simulink model "batt_test"  (Simulink 7.8)
settings: Solver=ode3  StartTime=0.0  StopTime=20  FixedStep=80e-6  RelTol=1e-3
PostLoadFcn:
  | Ts=80e-6;
InitFcn:
  | Ts=80e-6;
values from neighbouring files (symbols this model uses):
  batt_esr = (max_power*0.01)/(max_power/Vdc_nom)^2    [BES_init.m]
  C = IacRMS*18e-6    [BES_init.m]
  f = 60    [global_parameters.m]
  I_ki = 0.03    [BES_init.m]
  I_kp = 0.05    [BES_init.m]
  Iac_max = IGBT_currents(possible_currents(1))    [BES_init.m]
  Id_at_max = 3*max_pow*(2/3)/Vd_at_max    [BES_init.m]
  Iq_at_max = 3*max_pow*(2/3)/Vq_at_max    [BES_init.m]
  L = Vdc_nom/(IacRMS*0.2/(2/fs))    [BES_init.m]
  PLL_Ki = 0.001*30    (= 0.03)    [BES_init.m]
  PLL_Kp = .001*30    (= 0.03)    [BES_init.m]
  PLL_time_step = Ts    (= 8e-05)    [global_parameters.m]
  Roff = 1e7    (= 10000000)    [BES_init.m]
  Td_es_min = Ts    (= 8e-05)    [global_parameters.m]
  Tds = Ts    (= 8e-05)    [global_parameters.m]
  Vdc_max = IGBT_voltages(possible_voltages(1))    [BES_init.m]
undefined symbols (not defined in the file or in its folder): D, DiscIntNeverNeededParam
libraries: simulink x25, powerlib x20, simulink_extras x10, cstextras x9, powerlib_extras x8, modbus_lib x6, dynamic_load_lib x1, dspsigops x1
(part 1 of 2)
settings Model: Creator=ch24070  LastModifiedBy=ch24070

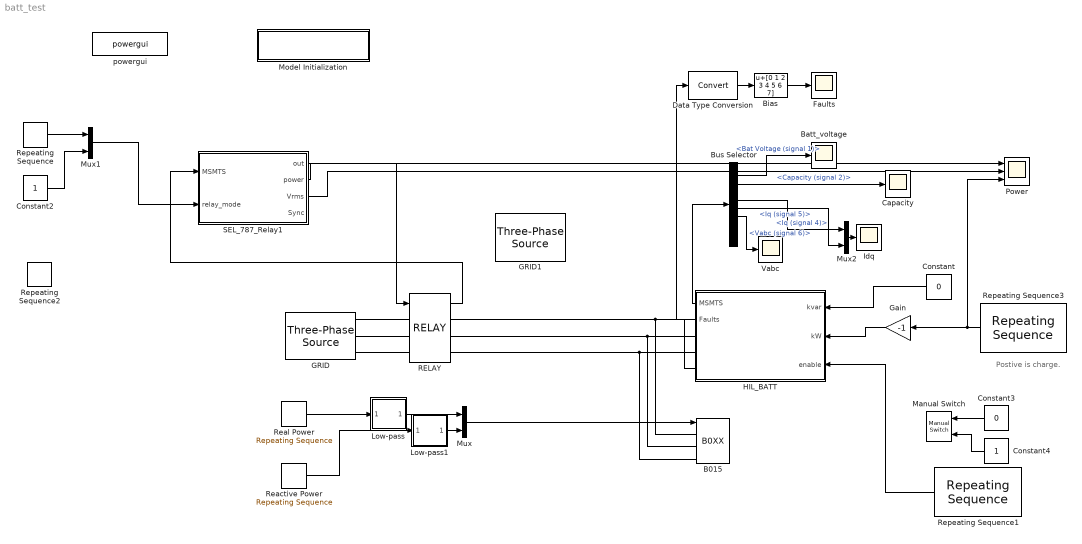
== system batt_test ==
  note: Postive is charge.
  B015 : dynamic_load_lib/B0XX  V=2047  P_Scale=1  Q_Scale=1
  Batt_voltage : Scope
      settings: YMin=500  YMax=4250  SaveName=ScopeData3
  Bias : Bias  Bias=[0 1 2 3 4 5 6 7]
  Bus Selector : BusSelector  OutputSignals=Bat Voltage (signal 1),Capacity (signal 2),Batt Iout (signal 3),Iq (signal 4),Iq (signal 5),Vabc (signal 6),Iabc (signal 7),freq (signal 8)
  Capacity : Scope
      settings: YMin=-0.05  YMax=1.05  SaveName=ScopeData4
  Constant : Constant  Value=0
  Constant2 : Constant
  Constant3 : Constant  Value=0
  Constant4 : Constant
  Data Type Conversion : DataTypeConversion
  Faults : Scope
      settings: TimeRange=10  YMin=0  YMax=10
  GRID : powerlib/Electrical Sources/Three-Phase Source  Voltage=2078  PhaseAngle=0  Frequency=60  InternalConnection=Yg  SpecifyImpedance=on  Resistance=0.8929  Inductance=16.58e-3  ShortCircuitLevel=375e6  BaseVoltage=2078  XRratio=7.9  BusType=swing  Pref=0  Qref=0  Qmin=-inf  Qmax=inf
  GRID1 : powerlib/Electrical Sources/Three-Phase Source  Voltage=1  PhaseAngle=0  Frequency=60*5  InternalConnection=Yg  SpecifyImpedance=on  Resistance=0.8929  Inductance=16.58e-3  ShortCircuitLevel=375e3  BaseVoltage=2078  XRratio=7.9  BusType=swing  Pref=0  Qref=0  Qmin=-inf  Qmax=inf
  Gain : Gain  Gain=-1
  HIL_BATT : Subsystem
  Idq : Scope
      settings: YMin=-1750  YMax=1750  SaveName=ScopeData6
  Low-pass : Subsystem  BlockChoice=CSS  mask(LTI Block){sys=c2d(tf(1,[1/(1*2*pi),1]),Ts), IC=[]}
      mask prompts: sys "LTI system variable"; IC "Initial states (state-space only)"
      mask help:
      | The LTI System block accepts both continuous and discrete LTI models as defined in the Control System Toolbox. Transfer function, state-space, and zero-pole-gain formats are all supported in this block.
      |
      | Note: Initial states are only meaningful for state-space systems.
      mask init:
      | try
      |    % read data to initialize mask variables
      |    [D,Ts,Tdi,Tdo,Tdio,x0,sysname]=...
      |       ltimask('Initialize',gcb,sys,IC);
      |    % update contents
      |    model = bdroot;
      |    df = get_param(model,'dirty');
      |    ltimask('UpdateDiagram',gcb,D,Ts,Tdio);
      |    try      
      |       % Attempt to modify locked library -> error
      |       % Makes block show ??? when loading CSTBLOCKS
      |       % for the first time
      |       set_param(model,'dirty',df)
      |    end
      | catch ME
      |    sys = [];  IC = [];   sysname = '???';
      |    throw(ME)
      | end
      mask Help:
      | The LTI System block accepts any of the three standard LTI models described in the Control System Toolbox: transfer function, zero/pole/gain, or state space. Internally, LTI models will be converted to their state space equivalent for evaluation.
      | <p>
      | In the editable text box labeled <b>LTI System Variable</b>, enter a valid LTI model.
      | <p>
      | In the editable text box labeled <b>Initial States</b> enter the initial state vector.  Initial states are only valid for state-space systems.
      | <p>
      | See also TF, ZPK, SS, LTIMODELS.
      mask CallbackString: ltimask('MaskLTICallback',gcb);|
      mask Display: disp(sysname)
  Low-pass1 : Subsystem  BlockChoice=CSS  mask(LTI Block){sys=c2d(tf(1,[1/(1*2*pi),1]),Ts), IC=[]}
      mask prompts: sys "LTI system variable"; IC "Initial states (state-space only)"
      mask help:
      | The LTI System block accepts both continuous and discrete LTI models as defined in the Control System Toolbox. Transfer function, state-space, and zero-pole-gain formats are all supported in this block.
      |
      | Note: Initial states are only meaningful for state-space systems.
      mask init: same as batt_test/Low-pass
      mask Help:
      | The LTI System block accepts any of the three standard LTI models described in the Control System Toolbox: transfer function, zero/pole/gain, or state space. Internally, LTI models will be converted to their state space equivalent for evaluation.
      | <p>
      | In the editable text box labeled <b>LTI System Variable</b>, enter a valid LTI model.
      | <p>
      | In the editable text box labeled <b>Initial States</b> enter the initial state vector.  Initial states are only valid for state-space systems.
      | <p>
      | See also TF, ZPK, SS, LTIMODELS.
      mask CallbackString: ltimask('MaskLTICallback',gcb);|
      mask Display: disp(sysname)
  Manual Switch : simulink/Signal Routing/Manual Switch  sw=1  action=0  varsize=off
  Model Initialization : Subsystem  AncestorBlock=artemis/Tools /Misc/Model Initialization  mask(Model Functions){InitFcnX=Ts=80e-6;, prel=off, posl=on, inif=on, strf=off}
      mask prompts: InitFcnX "Initialisation"; prel "Preload Function"; posl "PostLoad Function"; inif "InitFcn"; strf "StartFcn"
      mask init:
      | currentBlock = gcb;
      | root = bdroot(currentBlock);
      | 
      | if ~strcmp(get_param(root,'BlockDiagramType'),'library')
      |     if prel==1
      |         set_param(root, 'PreLoadFcn', InitFcnX);
      |     else
      |         set_param(root, 'PreLoadFcn', '');
      |     end
      |     if inif==1
      |         set_param(root, 'InitFcn', InitFcnX);
      |     else
      |         set_param(root, 'InitFcn', '');
      |     end
      |     if strf==1
      |         set_param(root, 'StartFcn', InitFcnX);
      |     else
      |         set_param(root, 'StartFcn', '');
      |     end
      |     if posl==1
      |         set_param(root, 'PostLoadFcn', InitFcnX);
      |     else
      |         set_param(root, 'PostLoadFcn', '');
      |     end
      | end
      | 
      | pos = get_param(currentBlock, 'Position');
      | width = pos(3) - pos(1); height = pos(4) - pos(2);
      | txt = [ upper(root) '\n' '- InitFcn. . . . . '  get_param(root, 'InitFcn') ];
      settings: CopyFcn=set_param(gcb,'LinkStatus','inactive')
      mask Display: text(5, height*0.5, txt, 'horizontalAlignment', 'left', 'verticalAlignment', 'middle') ;
  Mux : Mux  Inputs=2
  Mux1 : Mux  Inputs=2
  Mux2 : Mux  Inputs=2
  Power : Scope  NumInputPorts=3
      settings: YMin=-5000~0~3800  YMax=5000~1400~4200
  RELAY : modbus_lib/RELAY  Ts=Ts
      link override Three-Phase V-I Measurement/Model/VI/Ia: GotoTag=LibraryTag_Ia
      link override Three-Phase V-I Measurement/Model/VI/Ib: GotoTag=LibraryTag_Ib
      link override Three-Phase V-I Measurement/Model/VI/Ic: GotoTag=LibraryTag_Ic
      link override Three-Phase V-I Measurement/Model/VI/Va: GotoTag=LibraryTag_Va
      link override Three-Phase V-I Measurement/Model/VI/Vb: GotoTag=LibraryTag_Vb
      link override Three-Phase V-I Measurement/Model/VI/Vc: GotoTag=LibraryTag_Vc
      link override Three-Phase V-I Measurement1/Model/VI/Ia: GotoTag=LibraryTag_Ia
      link override Three-Phase V-I Measurement1/Model/VI/Ib: GotoTag=LibraryTag_Ib
      link override Three-Phase V-I Measurement1/Model/VI/Ic: GotoTag=LibraryTag_Ic
      link override Three-Phase V-I Measurement1/Model/VI/Va: GotoTag=LibraryTag_Va
      link override Three-Phase V-I Measurement1/Model/VI/Vb: GotoTag=LibraryTag_Vb
      link override Three-Phase V-I Measurement1/Model/VI/Vc: GotoTag=LibraryTag_Vc
  Reactive Power : simulink/Sources/Repeating Sequence  rep_seq_t=[0 2 4 6]  rep_seq_y=[0 50 0 50]
  Real Power : simulink/Sources/Repeating Sequence  rep_seq_t=[0 2 4 6]  rep_seq_y=[0 100 0 100]
  Repeating Sequence : simulink/Sources/Repeating Sequence  rep_seq_t=[0 2]  rep_seq_y=[0 0]
  Repeating Sequence1 : simulink/Sources/Repeating Sequence  rep_seq_t=[0 2 2 5 5 6 6 7 12]  rep_seq_y=[0 0 1 1 0 0 1 1 1]
  Repeating Sequence2 : simulink/Sources/Repeating Sequence  rep_seq_t=[0 3 3 5 5 6 7]  rep_seq_y=[0 0 2 2 1 1 0]
  Repeating Sequence3 : simulink/Sources/Repeating Sequence  rep_seq_t=[0 2 2 5 5 6 6 7 12]  rep_seq_y=4000.*[0 0 1 1 0 0 -1 -1 -1]
  SEL_787_Relay1 : Subsystem  mask{IOC=30000, TOC=2500, VRMSLL=13800, Ts=Ts}
      mask prompts: IOC "IOC Setting [A]"; TOC "TOC Setting [A]"; VRMSLL "Nominal Voltage [VRMSLL]"; Ts "Sampling Time [Sec]"
  Vabc : Scope
      settings: TimeRange=5.446467479375272e-005  YMin=-0.02823442247358754  YMax=0.1118314007674113  SaveName=ScopeData2
  powergui : powerlib/powergui  Priority=2  SimulationMode=Discrete  SolverType=Tustin  SampleTime=Ts  frequency=60  SPID=off  DisableSnubberDevices=off  DisableRonSwitches=off  DisableVfSwitches=off  SwTol=0  Interpol=off  DisplayEquations=off  FunctionMessages=off  frequencyindice=0  Pbase=100e6  ErrMax=1e-4  Iterations=50  UnitsV=kV  UnitsW=MW  echomessages=off  HookPort=off  EnableUseOfTLC=off  x0status=blocks  RestoreLinks=warning  ResistiveCurrentMeasurement=off  Frange=logspace(0,3,50)  Ylog=off  Xlog=off  ShowGrid=off  save=off  variable=ZData  structure=0  ZoomFFT=on  StartTime=0.0  cycles=2  DisplayStyle=off  fundamental=60  FreqAxis=off  MaxFrequency=1000  frequencyindicesteady=1  RmsSteady=1  display=off  Ts=0  methode=off
  wires:
  RELAY/1 -> SEL_787_Relay1/1(MSMTS)
  HIL_BATT/1(MSMTS) -> Bus Selector/1
  HIL_BATT/2(Faults) -> Data Type Conversion/1
  Constant/1 -> HIL_BATT/1(kvar)
  Repeating Sequence3/1 -> Gain/1, Power/3
  SEL_787_Relay1/1(out) -> RELAY/1
  SEL_787_Relay1/2(power) -> Power/1
  Bus Selector/6 -> Vabc/1  "<Vabc (signal 6)>"
  Bus Selector/1 -> Batt_voltage/1  "<Bat Voltage (signal 1)>"
  Bus Selector/2 -> Capacity/1  "<Capacity (signal 2)>"
  Gain/1 -> HIL_BATT/2(kW)
  Bias/1 -> Faults/1
  Data Type Conversion/1 -> Bias/1
  Mux/1 -> B015/1
  Real Power/1 -> Low-pass/1(In1)
  Reactive Power/1 -> Low-pass1/1(In1)
  Low-pass/1(Out1) -> Mux/1
  Low-pass1/1(Out1) -> Mux/2
  Mux1/1 -> SEL_787_Relay1/2(relay_mode)
  SEL_787_Relay1/3(Vrms) -> Power/2
  Repeating Sequence/1 -> Mux1/1
  Constant2/1 -> Mux1/2
  Constant3/1 -> Manual Switch/1
  Constant4/1 -> Manual Switch/2
  Mux2/1 -> Idq/1
  Bus Selector/4 -> Mux2/1  "<Iq (signal 4)>"
  Bus Selector/5 -> Mux2/2  "<Iq (signal 5)>"
  Repeating Sequence1/1 -> HIL_BATT/3(enable)
  connections:
  GRID/RConn2 -- RELAY/LConn2
  GRID/RConn1 -- RELAY/LConn1
  GRID/RConn3 -- RELAY/LConn3
  RELAY/RConn1 -- HIL_BATT/RConn1 -- B015/LConn1
  RELAY/RConn2 -- HIL_BATT/RConn2 -- B015/LConn2
  RELAY/RConn3 -- HIL_BATT/RConn3 -- B015/LConn3

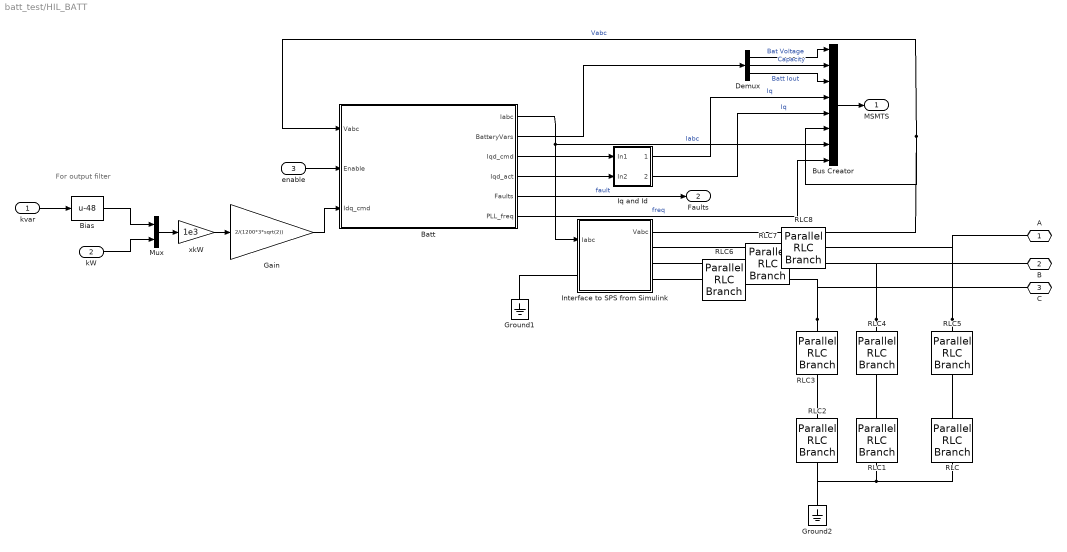
== system batt_test/HIL_BATT ==
  note: For output filter
  kvar : Inport
  kW : Inport  Port=2
  enable : Inport  Port=3
  Batt : Subsystem  mask(Battery Energy Storage System with AC inverter and Droop Control){max_power=4e6, batt_kWh=5, VacRMS=1200, Vdc_nom=4000}
      mask prompts: max_power "Peak Power (W)"; batt_kWh "Capacity (kWh)"; VacRMS "Grid Tie Line to Neutral Voltage (RMS)"; Vdc_nom "Nominal DC Battery Voltage"
      mask help: The block implements a battery energy storage system suitable for connecting to the grid. It responds to grid voltage changes by injecting current into the grid. The model is a non-switching average model.
      mask init:
      | global_parameters
      | BES_init
      mask Help:
      | This block will likely need a filter and transformer on it's output in order to connect to a high power line.
      | 
      | A unit delay block  on the Iabc output can help remove algebraic loops with minimal impact on simulation results.
      | 
      | 
      | Block Parameters:
      | Peak Power- Maximum power the unit can transfer.
      | Capacity- Amount of energy in the battery.
      | Grid Tie Line to Neutral Voltage- RMS voltage for the grid tie interface.
      | Nominal DC Battery Voltage- Open circuit full charge voltage.
      | Real Power Droop Gain- Ratio of Watts to Hz for injecting power to the grid in response to frequency changes.
      | Reactive Power Droop Gain- Ratio of kVars to RMS volts for injecting reactive power to the grid.
      | Droop Filter Cut Off- Fastest frequency that will be responded to for injecting power to the grid.
      | 
      | 
      | Block Connections:
      | Vabc- Grid voltage for each of the three phases.
      | Enable- Set to zero for no power.  Set to 1 to enable energy tranfer.
      | Iabc- Grid current for each of the three phases.  Connect to your grid.  Positive is into the grid.
      | Battery_vars- A vector of battery voltage, capacity, and current out of the battery.
      | Iqd_cmd- Commanded q and d axis currents.
      | Iqd_act- Actual q and d axis currents.
      mask Display:
      | image(imread('grid_storage_battery.jpg'))
      | color('white')
      | fprintf('%d kW Peak', max_power/1e3)
      | color('black')
      | port_label('input',1,'Vabc')
      | port_label('input',2,'Enable')
      | port_label('input',3,'Idq_cmd')
      | port_label('output',1,'Iabc')
      | port_label('output',2,'Battery_vars')
      | port_label('output',3,'Iqd_cmd')
      | port_label('output',4,'Iqd_act')
      | port_label('output',5,'Faults')
      | port_label('output',6,'Freq')
  Bias : Bias  Bias=-48
  Bus Creator : BusCreator  Inputs=8
  Demux : Demux  Outputs=3
  Gain : Gain  Gain=2/(1200*3*sqrt(2))
  Ground1 : powerlib/Elements/Ground  LConnTagsString=a
  Ground2 : powerlib/Elements/Ground  LConnTagsString=a
  Interface to SPS from Simulink : Subsystem
  Iq and Id : Subsystem
  Mux : Mux  Inputs=2
  "RLC " : powerlib/Elements/Parallel RLC Branch  LConnTagsString=a  RConnTagsString=__new0  BranchType=RLC  Resistance=500  Inductance=inf  SetiL0=off  InitialCurrent=0  Capacitance=10e-6  Setx0=off  InitialVoltage=0  Measurements=None
  RLC1 : powerlib/Elements/Parallel RLC Branch  LConnTagsString=a  RConnTagsString=__new0  BranchType=RLC  Resistance=500  Inductance=inf  SetiL0=off  InitialCurrent=0  Capacitance=10e-6  Setx0=off  InitialVoltage=0  Measurements=None
  RLC2 : powerlib/Elements/Parallel RLC Branch  LConnTagsString=a  RConnTagsString=__new0  BranchType=RLC  Resistance=500  Inductance=inf  SetiL0=off  InitialCurrent=0  Capacitance=10e-6  Setx0=off  InitialVoltage=0  Measurements=None
  RLC3 : powerlib/Elements/Parallel RLC Branch  LConnTagsString=a  RConnTagsString=__new0  BranchType=R  Resistance=10e-3  Inductance=inf  SetiL0=off  InitialCurrent=0  Capacitance=0  Setx0=off  InitialVoltage=0  Measurements=None
  RLC4 : powerlib/Elements/Parallel RLC Branch  LConnTagsString=a  RConnTagsString=__new0  BranchType=R  Resistance=10e-3  Inductance=inf  SetiL0=off  InitialCurrent=0  Capacitance=0  Setx0=off  InitialVoltage=0  Measurements=None
  RLC5 : powerlib/Elements/Parallel RLC Branch  LConnTagsString=a  RConnTagsString=__new0  BranchType=R  Resistance=10e-3  Inductance=inf  SetiL0=off  InitialCurrent=0  Capacitance=0  Setx0=off  InitialVoltage=0  Measurements=None
  RLC6 : powerlib/Elements/Parallel RLC Branch  LConnTagsString=a  RConnTagsString=__new0  BranchType=R  Resistance=20e-3  Inductance=inf  SetiL0=off  InitialCurrent=0  Capacitance=0  Setx0=off  InitialVoltage=0  Measurements=None
  RLC7 : powerlib/Elements/Parallel RLC Branch  LConnTagsString=a  RConnTagsString=__new0  BranchType=R  Resistance=20e-3  Inductance=inf  SetiL0=off  InitialCurrent=0  Capacitance=0  Setx0=off  InitialVoltage=0  Measurements=None
  RLC8 : powerlib/Elements/Parallel RLC Branch  LConnTagsString=a  RConnTagsString=__new0  BranchType=R  Resistance=20e-3  Inductance=inf  SetiL0=off  InitialCurrent=0  Capacitance=0  Setx0=off  InitialVoltage=0  Measurements=None
  xkW : Gain  Gain=1e3
  A : PMIOPort  Port=1  Side=Right
  B : PMIOPort  Port=2  Side=Right
  C : PMIOPort  Port=3  Side=Right
  MSMTS : Outport
  Faults : Outport  Port=2
  wires:
  Bias/1 -> Mux/1
  Batt/6(PLL_freq) -> Bus Creator/8  "freq"
  kW/1 -> Mux/2
  kvar/1 -> Bias/1
  Bus Creator/1 -> MSMTS/1
  Iq and Id/2(Out2) -> Bus Creator/5  "Iq"
  Mux/1 -> xkW/1
  xkW/1 -> Gain/1
  Gain/1 -> Batt/3(Idq_cmd)
  Batt/1(Iabc) -> Interface to SPS from Simulink/1(Iabc), Bus Creator/7  "Iabc"
  enable/1 -> Batt/2(Enable)
  Iq and Id/1(Out1) -> Bus Creator/4  "Iq"
  Batt/4(Iqd_act) -> Iq and Id/2(In2)
  Batt/3(Iqd_cmd) -> Iq and Id/1(In1)
  Demux/1 -> Bus Creator/1  "Bat Voltage"
  Demux/3 -> Bus Creator/3  "Batt Iout"
  Demux/2 -> Bus Creator/2  "Capacity"
  Batt/2(BatteryVars) -> Demux/1
  Interface to SPS from Simulink/1(Vabc) -> Bus Creator/6, Batt/1(Vabc)  "Vabc"
  Batt/5(Faults) -> Faults/1  "fault"
  connections:
  Interface to SPS from Simulink/RConn1 -- RLC8/RConn1
  Interface to SPS from Simulink/RConn2 -- RLC7/RConn1
  RLC6/RConn1 -- Interface to SPS from Simulink/RConn3
  RLC5/RConn1 -- "RLC "/LConn1
  RLC4/RConn1 -- RLC1/LConn1
  RLC3/RConn1 -- RLC2/LConn1
  RLC3/LConn1 -- RLC6/LConn1 -- C/RConn1
  RLC4/LConn1 -- RLC7/LConn1 -- B/RConn1
  RLC5/LConn1 -- RLC8/LConn1 -- A/RConn1
  RLC1/RConn1 -- "RLC "/RConn1 -- RLC2/RConn1 -- Ground2/LConn1
  Interface to SPS from Simulink/LConn1 -- Ground1/LConn1

== system batt_test/Low-pass ==
  In1 : Inport
  IO Delay : cstextras/Integer Delay (masked)  Td=Tdio  u0=0  Ts=Ts
  Input Delay : cstextras/Integer Delay (masked)  Td=Tdi  u0=0  Ts=Ts
  Internal : DiscreteStateSpace  A=D.a  B=D.b  C=D.c  D=D.d  SampleTime=Ts
  Output Delay : cstextras/Integer Delay (masked)  Td=Tdo  u0=0  Ts=Ts
  Out1 : Outport  InitialOutput=0
  wires:
  In1/1 -> Input Delay/1
  Output Delay/1 -> Out1/1
  Input Delay/1 -> Internal/1
  Internal/1 -> IO Delay/1
  IO Delay/1 -> Output Delay/1

== system batt_test/Low-pass1 ==
  In1 : Inport
  IO Delay : cstextras/Integer Delay (masked)  Td=Tdio  u0=0  Ts=Ts
  Input Delay : cstextras/Integer Delay (masked)  Td=Tdi  u0=0  Ts=Ts
  Internal : DiscreteStateSpace  A=D.a  B=D.b  C=D.c  D=D.d  SampleTime=Ts
  Output Delay : cstextras/Integer Delay (masked)  Td=Tdo  u0=0  Ts=Ts
  Out1 : Outport  InitialOutput=0
  wires:
  In1/1 -> Input Delay/1
  Output Delay/1 -> Out1/1
  Input Delay/1 -> Internal/1
  Internal/1 -> IO Delay/1
  IO Delay/1 -> Output Delay/1

== system batt_test/Model Initialization ==

== system batt_test/SEL_787_Relay1 ==
  MSMTS : Inport
  relay_mode : Inport  Port=2
  Bus Creator : BusCreator  Inputs=3
  Bus Selector1 : BusSelector  OutputSignals=Iabc,Vabc_bus,Vabc_line
  Bus Selector2 : BusSelector  OutputSignals=signal19,signal20,signal10
  Mux : Mux  Inputs=2
  SEL_787_Relay : Subsystem  AncestorBlock=modbus_lib/SEL_787_Relay  mask(SEL_787){bkrCtrl_enable=0, bkrCtrl_status=1}
      mask prompts: bkrCtrl_enable "Enable - manual breaker control"; bkrCtrl_status "Status - manual breaker control"
      mask help:
      | Reynaldo Ulerio
      | Jason LaPenta
      | Aidan Dowdle
      | Matt Backes
      | Sept 14, 2015
      | ________________________________
      |
      | Based off the SEL-787 transformer relay, this model receives
      | the three-phase current and voltage measurements, and packs
      | them along with other calculations to send to the microgrid
      | controller via Modbus
      |
      | - See HIL packet for detailed list of signals and scale factors
      | - Follows convention of IEEE C37.2-2008
      |
      | Procedure to reclose a breaker:
      | 1) reset all relay functions
      | 2) set orvvp_mode==1 to force breaker to close
      |    --> The relay function 25 will automatically activate
      | 3) change op_mode==0 for logic based operation
      |
      | * Additional and for debuging: Allows the user to select which trip signal will be received at the breaker.
      |
      | Manual breaker status: [1-closed, 0-open]
  out : Outport
  power : Outport  Port=2
  Vrms : Outport  Port=3
  Sync : Outport  Port=4
  wires:
  SEL_787_Relay/1(op_mode) -> Bus Creator/1  "op_mode"
  SEL_787_Relay/2(Logic_trip) -> Bus Creator/2  "Logic_trip"
  SEL_787_Relay/3(m) -> Bus Creator/3  "m"
  SEL_787_Relay/4(TO_MODBUS) -> Bus Selector2/1
  Bus Creator/1 -> out/1  "SEL_787_Relay1"
  MSMTS/1 -> Bus Selector1/1
  Bus Selector1/1 -> SEL_787_Relay/1(Iabc)  "<Iabc>"
  Bus Selector1/2 -> SEL_787_Relay/2(Vabc_bus)  "<Vabc_bus>"
  Bus Selector1/3 -> SEL_787_Relay/3(Vabc_line)  "<Vabc_line>"
  Bus Selector2/1 -> Mux/1  "<signal19>"
  Bus Selector2/2 -> Mux/2  "<signal20>"
  Mux/1 -> power/1
  relay_mode/1 -> SEL_787_Relay/4(FROM_MODBUS)
  Bus Selector2/3 -> Vrms/1  "<signal10>"
  SEL_787_Relay/5(Sync) -> Sync/1

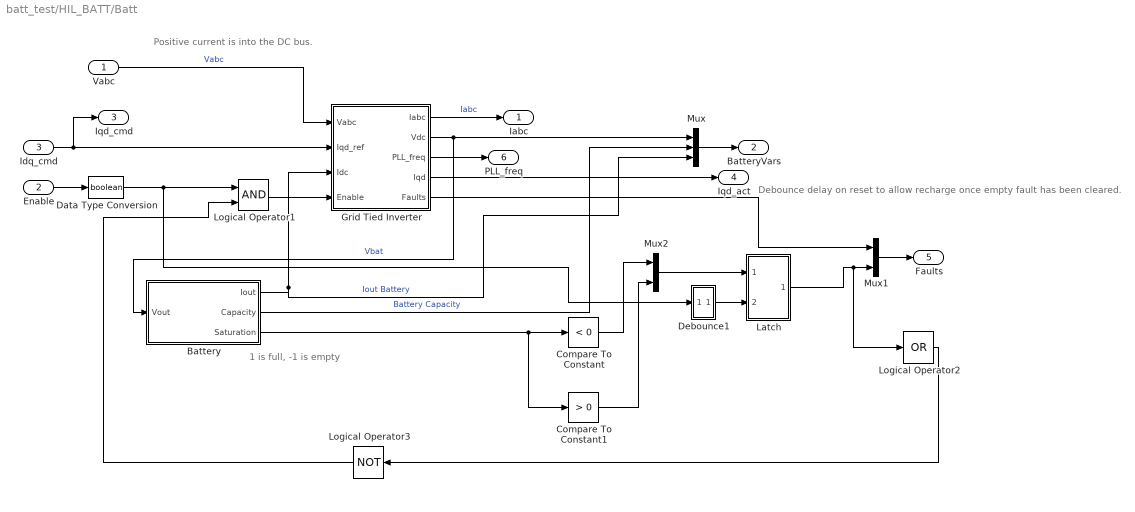
== system batt_test/HIL_BATT/Batt ==
  note: Positive current is into the DC bus.
  note: 1 is full, -1 is empty
  note: Debounce delay on reset to allow recharge once empty fault has been cleared.
  Vabc : Inport
  Enable : Inport  Port=2  OutDataTypeStr=double
  Idq_cmd : Inport  Port=3
  Battery : Subsystem  mask(Very simple battery model.  ){kWh=batt_kWh, esr=batt_esr, Vdc_nom=Vdc_nom}
      mask prompts: kWh "Capacity  (kWh)"; esr "Output Resistance (Ohms)"; Vdc_nom "Open Circuit Voltage"
      mask help: Model integrates charge and stops at the rated capacity. When charge is all removed the current drops to zero.
      mask Help: This model views the battery as a voltage source with a fixed equivalent series resistance and a perfect integrator for capacity.
  Compare To Constant : simulink/Logic and Bit Operations/Compare To Constant  relop=<  const=0  OutDataTypeStr=boolean
  Compare To Constant1 : simulink/Logic and Bit Operations/Compare To Constant  relop=>  const=0  OutDataTypeStr=boolean
  Data Type Conversion : DataTypeConversion  OutDataTypeStr=boolean
  Debounce1 : Subsystem  mask{Ts=Ts, Td=0.1}
      mask prompts: Ts "Sample Time"; Td "Debounce Time"
  Grid Tied Inverter : Subsystem
  Latch : Subsystem
  Logical Operator1 : Logic  AllPortsSameDT=off  OutDataTypeStr=boolean
  Logical Operator2 : Logic  Operator=OR  Inputs=1  AllPortsSameDT=off  OutDataTypeStr=boolean
  Logical Operator3 : Logic  Operator=NOT  AllPortsSameDT=off  OutDataTypeStr=boolean
  Mux : Mux  Inputs=3
  Mux1 : Mux  Inputs=2
  Mux2 : Mux  Inputs=2
  Iabc : Outport
  BatteryVars : Outport  Port=2
  Iqd_cmd : Outport  Port=3
  Iqd_act : Outport  Port=4
  Faults : Outport  Port=5
  PLL_freq : Outport  Port=6
  wires:
  Grid Tied Inverter/3(PLL_freq) -> PLL_freq/1
  Vabc/1 -> Grid Tied Inverter/1(Vabc)  "Vabc"
  Grid Tied Inverter/2(Vdc) -> Mux/1, Battery/1(Vout)  "Vbat"
  Battery/1(Iout) -> Grid Tied Inverter/3(Idc), Mux/3  "Iout Battery"
  Battery/2(Capacity) -> Mux/2  "Battery Capacity"
  Grid Tied Inverter/1(Iabc) -> Iabc/1  "Iabc"
  Mux/1 -> BatteryVars/1
  Grid Tied Inverter/4(Iqd) -> Iqd_act/1
  Idq_cmd/1 -> Grid Tied Inverter/2(Iqd_ref), Iqd_cmd/1
  Enable/1 -> Data Type Conversion/1
  Mux1/1 -> Faults/1
  Battery/3(Saturation) -> Compare To Constant/1, Compare To Constant1/1
  Compare To Constant/1 -> Mux2/1
  Compare To Constant1/1 -> Mux2/2
  Logical Operator1/1 -> Grid Tied Inverter/4(Enable)
  Data Type Conversion/1 -> Logical Operator1/1, Debounce1/1(In1)
  Logical Operator2/1 -> Logical Operator3/1
  Logical Operator3/1 -> Logical Operator1/2
  Grid Tied Inverter/5(Faults) -> Mux1/1
  Latch/1(Out1) -> Mux1/2, Logical Operator2/1
  Mux2/1 -> Latch/1(In1)
  Debounce1/1(Out1) -> Latch/2(Reset)

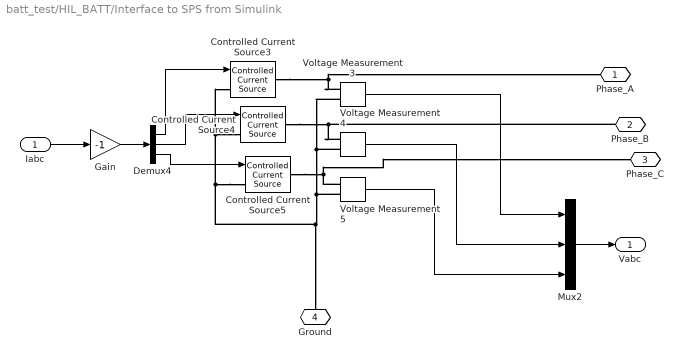
== system batt_test/HIL_BATT/Interface to SPS from Simulink ==
  Iabc : Inport
  Controlled Current Source3 : powerlib/Electrical Sources/Controlled Current Source  Initialize=on  Source_Type=AC  Amplitude=0  Phase=0  Frequency=0  Measurements=None
  Controlled Current Source4 : powerlib/Electrical Sources/Controlled Current Source  Initialize=on  Source_Type=AC  Amplitude=0  Phase=0  Frequency=0  Measurements=None
  Controlled Current Source5 : powerlib/Electrical Sources/Controlled Current Source  Initialize=on  Source_Type=AC  Amplitude=0  Phase=0  Frequency=0  Measurements=None
  Demux4 : Demux  Outputs=3
  Gain : Gain  Gain=-1
  Mux2 : Mux  Inputs=3
  Voltage Measurement3 : powerlib/Measurements/Voltage Measurement  PhasorSimulation=off  OutputType=Complex  PSBequivalent=0
  Voltage Measurement4 : powerlib/Measurements/Voltage Measurement  PhasorSimulation=off  OutputType=Complex  PSBequivalent=0
  Voltage Measurement5 : powerlib/Measurements/Voltage Measurement  PhasorSimulation=off  OutputType=Complex  PSBequivalent=0
  Phase_A : PMIOPort  Port=1  Side=Right
  Phase_B : PMIOPort  Port=2  Side=Right
  Phase_C : PMIOPort  Port=3  Side=Right
  Ground : PMIOPort  Port=4  Side=Left
  Vabc : Outport
  wires:
  Voltage Measurement5/1 -> Mux2/3
  Voltage Measurement4/1 -> Mux2/2
  Demux4/1 -> Controlled Current Source3/1
  Demux4/2 -> Controlled Current Source4/1
  Demux4/3 -> Controlled Current Source5/1
  Iabc/1 -> Gain/1
  Mux2/1 -> Vabc/1
  Voltage Measurement3/1 -> Mux2/1
  Gain/1 -> Demux4/1
  connections:
  Voltage Measurement5/LConn1 -- Controlled Current Source5/RConn1 -- Phase_C/RConn1
  Voltage Measurement3/LConn1 -- Controlled Current Source3/RConn1 -- Phase_A/RConn1
  Controlled Current Source5/LConn1 -- Controlled Current Source3/LConn1 -- Controlled Current Source4/LConn1 -- Voltage Measurement4/LConn2 -- Voltage Measurement3/LConn2 -- Voltage Measurement5/LConn2 -- Ground/RConn1
  Voltage Measurement4/LConn1 -- Controlled Current Source4/RConn1 -- Phase_B/RConn1

== system batt_test/HIL_BATT/Iq and Id ==
  In1 : Inport
  In2 : Inport  Port=2
  Demux1 : Demux  Outputs=2
  Demux2 : Demux  Outputs=2
  Mux : Mux  Inputs=2
  Mux1 : Mux  Inputs=2
  Out1 : Outport
  Out2 : Outport  Port=2
  wires:
  Mux1/1 -> Out2/1
  Mux/1 -> Out1/1
  In2/1 -> Demux2/1
  In1/1 -> Demux1/1
  Demux2/2 -> Mux1/2  "Id_act"
  Demux1/1 -> Mux/1  "Iq_cmd"
  Demux2/1 -> Mux/2  "Iq_act"
  Demux1/2 -> Mux1/1  "Id_cmd"

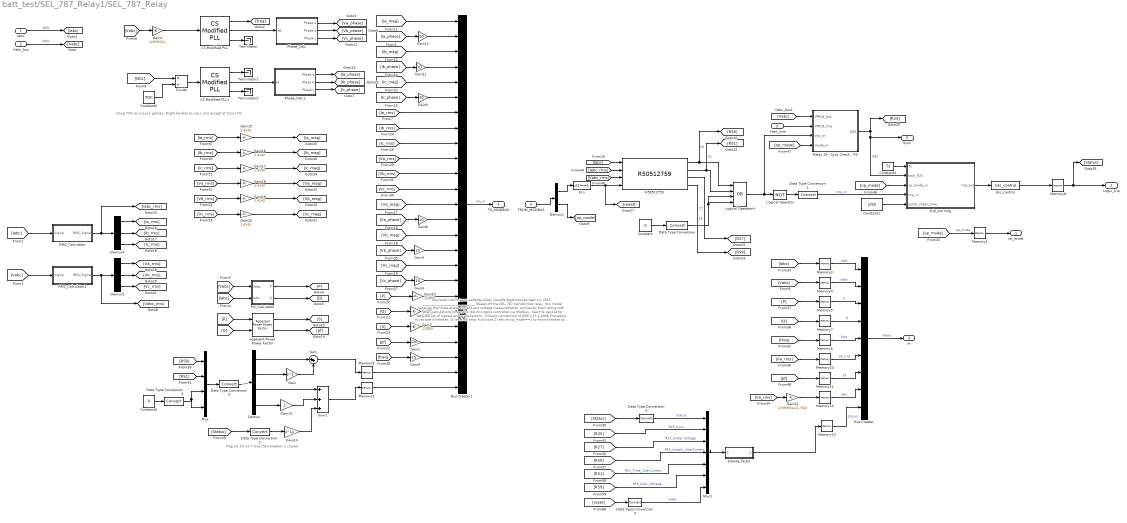
== system batt_test/SEL_787_Relay1/SEL_787_Relay ==
  note: Reg 24: bit 14 = true then breaker is closed
  note: Using TOC as a quick getway. Might be able to use I_rms except at time t=0.
  note: Reynaldo Ulerio
      | Jason LaPenta
      | Aidan Dowdle
      | Matt Backes
      | Sept 14, 2015
      | ________________________________
      |
      | Based off the SEL-787 transformer relay, this model receives
      | the three-phase current and voltage measurements, and packs
      | them along with other calculations to send to the microgrid
      | controller via Modbus
      |
      | - See HIL packet for detailed list of signals and scale factors
      | - Follows convention of IEEE C37.2-2008
      |
      | Procedure to reclose a breaker:
      | 1) reset all relay functions
      | 2) set orvvp_mode==1 to force breaker to close
      |    --> The relay function 25 will automatically activate
      | 3) change op_mode==0 for logic based operation
  Iabc : Inport
  Vabc_bus : Inport  Port=2
  Vabc_line : Inport  Port=3
  FROM_MODBUS : Inport  Port=4
  Apparent Power Power Factor : modbus_lib/Apparent Power Power Factor
  Bus Creator : BusCreator  Inputs=9
  Bus Creator1 : BusCreator  Inputs=25
  CS Modified PLL : modbus_lib/CS Modified PLL  Fmin=50  Par_Init=[0 60]  ParK=[ 180 3200 1 ]  Ts=Ts  AGC=off
  CS Modified PLL1 : modbus_lib/CS Modified PLL  Fmin=50  Par_Init=[0 60]  ParK=[ 180 3200 1 ]  Ts=Ts  AGC=off
  Constant : Constant  Value=0
  Constant1 : Constant  Value=2/60
  Constant2 : Constant  Value=TOC
  Constant3 : Constant  Value=0
  Constant4 : Constant  Value=Ts
  Data Type Conversion{,1..6} (7 alike) : DataTypeConversion
  Demux : Demux
  Demux2 : Demux  Outputs=2
  Demux4 : Demux  Outputs=3
  Demux5 : Demux  Outputs=3
  Divide : Product  Inputs=*/
  Fcn : Fcn  Expr=u(1)==1
  Gain : Gain  Gain=2^3
  Gain1 : Gain  Gain=100
  Gain10 : Gain  Gain=1/1000
  Gain{3..5,8..9,11..12} (7 alike) : Gain  Gain=10
  Gain13 : Gain  Gain=2
  Gain14 : Gain  Gain=2^14
  Gain{15..20} (6 alike) : Gain  Gain=1.4142
  Gain2 : Gain  Gain=1/VRMSLL
  Gain21 : Gain  Gain=1/(VRMSLL/1.732)
  Gain6 : Gain  Gain=1/1000
  Gain7 : Gain  Gain=1/1000
  Logical Operator : Logic  Operator=NOT  AllPortsSameDT=off  OutDataTypeStr=boolean
  Logical Operator4 : Logic  Operator=OR  Inputs=4  AllPortsSameDT=off  OutDataTypeStr=boolean
  Memory{1..13} (13 alike) : Memory
  Mux : Mux
  Mux1 : Mux  Inputs=7
  PQ_Calculator : Subsystem
  Phase_Calc : Subsystem
  Phase_Calc1 : Subsystem
  R50512759 : modbus_lib/R50512759  VRMSLL=VRMSLL  IOC=IOC  TOC=TOC  Ts=Ts
  RMS_Calculator : Subsystem
  RMS_Calculator1 : Subsystem
  Relay 25 - Sync Check - RS : Subsystem  AncestorBlock=modbus_lib/Relay 25 - Sync Check - RS  mask{VRMSLL=VRMSLL, Ts=Ts}
      mask prompts: VRMSLL "Nominal Voltage [VRMSLL]"; Ts "Sampling Time [Sec]"
  Sum : Sum  Inputs=|++
  Sum1 : Sum  Inputs=+++
  Terminator : Terminator
  Terminator1 : Terminator
  Terminator2 : Terminator
  bitwise_faults : Subsystem
  bkr_control : modbus_lib/bkr_control  enable=bkrCtrl_enable  status=bkrCtrl_status
  trip_out mng : MATLAB Function  TreatAsAtomicUnit=on
  op_mode : Outport
  Logic_trip : Outport  Port=2
  m : Outport  Port=3
  TO_MODBUS : Outport  Port=4
  Sync : Outport  Port=5
  wires:
  Data Type Conversion6/1 -> Mux1/1  "Status"
  Data Type Conversion5/1 -> Mux1/7  "reset"
  [R59] -> Mux1/6  "R59_Over_Voltage"
  [R51] -> Mux1/5  "R51_Time_OverCurrent"
  [R50] -> Mux1/4  "R50_Instant_OverCurrent"
  [R27] -> Mux1/3  "R27_Under Voltage"
  [R25] -> Mux1/2  "R25_Sync"
  [Status] -> Data Type Conversion6/1
  [reset] -> Data Type Conversion5/1
  bitwise_faults/1(s) -> Memory13/1
  Mux1/1 -> bitwise_faults/1(S)
  Data Type Conversion3/1 -> Mux/4, Mux/3
  Constant3/1 -> Data Type Conversion3/1
  R50512759/4 -> [R59]  "59"
  R50512759/3 -> [R27]  "27"
  Data Type Conversion/1 -> Logical Operator4/3, Logical Operator4/4
  Constant/1 -> Data Type Conversion/1
  bkr_control/1 -> Memory8/1
  Bus Creator/1 -> m/1  "meas"
  Memory13/1 -> Bus Creator/9  "status"
  Apparent Power Power Factor/2 -> [pf]
  Apparent Power Power Factor/1 -> [S]
  Constant4/1 -> trip_out mng/1(Ts)
  Gain21/1 -> Memory12/1
  Memory12/1 -> Bus Creator/8  "Vpu"
  [Va_rms] -> Gain21/1
  Gain15/1 -> [Ia_mag]
  Gain16/1 -> [Ib_mag]
  Gain17/1 -> [Ic_mag]
  Gain18/1 -> [Va_mag]
  Gain19/1 -> [Vb_mag]
  Gain20/1 -> [Vc_mag]
  [Vc_rms] -> Gain20/1
  [Vb_rms] -> Gain19/1
  [Va_rms] -> Gain18/1
  [Ic_rms] -> Gain17/1
  [Ib_rms] -> Gain16/1
  [Ia_rms] -> Gain15/1
  Vabc_bus/1 -> [Vabc]  "Vabc"
  Vabc_line/1 -> Relay 25 - Sync Check - RS/2(VPKLN_line)
  [Vabc] -> Relay 25 - Sync Check - RS/1(VPKLN_bus)
  [Status] -> Data Type Conversion2/1
  Gain14/1 -> Sum1/3
  Data Type Conversion2/1 -> Gain14/1
  Gain4/1 -> Bus Creator1/23
  Gain1/1 -> Bus Creator1/22
  Gain7/1 -> Bus Creator1/21
  Gain6/1 -> Bus Creator1/20
  Gain10/1 -> Bus Creator1/19
  Gain3/1 -> Bus Creator1/18
  [Vc_mag] -> Bus Creator1/17
  Gain5/1 -> Bus Creator1/16
  [Vb_mag] -> Bus Creator1/15
  Gain8/1 -> Bus Creator1/14
  [Va_mag] -> Bus Creator1/13
  [Vc_rms] -> Bus Creator1/12
  [Vb_rms] -> Bus Creator1/11
  [Va_rms] -> Bus Creator1/10
  [Ic_rms] -> Bus Creator1/9
  [Ib_rms] -> Bus Creator1/8
  [Ia_rms] -> Bus Creator1/7
  Gain9/1 -> Bus Creator1/6
  [Ic_mag] -> Bus Creator1/5
  Gain11/1 -> Bus Creator1/4
  [Ib_mag] -> Bus Creator1/3
  Gain12/1 -> Bus Creator1/2
  [Ia_mag] -> Bus Creator1/1
  Memory11/1 -> Bus Creator/7  "pf"
  [pf] -> Memory11/1
  Memory10/1 -> Bus Creator/6  "Va_rms"
  Memory6/1 -> Bus Creator/5  "freq"
  [Va_rms] -> Memory10/1
  [freq] -> Memory6/1
  CS Modified PLL/3 -> Terminator/1
  CS Modified PLL1/3 -> Terminator2/1
  CS Modified PLL1/1 -> Terminator1/1
  CS Modified PLL/2 -> Phase_Calc/1(wt)
  CS Modified PLL/1 -> [freq]
  CS Modified PLL1/2 -> Phase_Calc1/1(wt)
  trip_out mng/1(trip_out) -> bkr_control/1
  [op_mode] -> Relay 25 - Sync Check - RS/4(mode_in)
  Data Type Conversion1/1 -> trip_out mng/4(trip_in)  "trip_in"
  [op_mode] -> trip_out mng/3(op_mode_in)
  Relay 25 - Sync Check - RS/1(R25) -> [R25], trip_out mng/2(bool_R25), Sync/1  "R25"
  Constant1/1 -> trip_out mng/5(synch_check_time)
  Memory8/1 -> [Status], Logic_trip/1
  Memory1/1 -> op_mode/1
  [op_mode] -> Memory1/1  "op_mode"
  Fcn/1 -> [reset], R50512759/4
  [Iabc_rms] -> R50512759/2
  Memory7/1 -> Bus Creator/4  "Q"
  Memory5/1 -> Bus Creator/3  "P"
  Memory4/1 -> Bus Creator/2  "Vabc"
  Memory3/1 -> Bus Creator/1  "Iabc"
  Memory2/1 -> Bus Creator1/25
  Memory9/1 -> Bus Creator1/24
  Data Type Conversion4/1 -> Demux/1
  Demux/4 -> Gain13/1
  Demux/3 -> Sum1/1
  Demux/2 -> Gain/1
  Demux/1 -> Sum/1
  Mux/1 -> Data Type Conversion4/1
  [R51] -> Mux/2
  [R50] -> Mux/1
  R50512759/2 -> [R51], Logical Operator4/2  "51"
  Gain/1 -> Sum/2
  Sum/1 -> Memory9/1
  Gain13/1 -> Sum1/2
  Sum1/1 -> Memory2/1
  R50512759/1 -> [R50], Logical Operator4/1  "50"
  Logical Operator/1 -> Data Type Conversion1/1
  Logical Operator4/1 -> Relay 25 - Sync Check - RS/3(trip_or), Logical Operator/1
  [Vabc_rms] -> R50512759/3
  [Ia_phase] -> Gain12/1
  [Ib_phase] -> Gain11/1
  [Ic_phase] -> Gain9/1
  [Va_phase] -> Gain8/1
  [Vb_phase] -> Gain5/1
  [Vc_phase] -> Gain3/1
  Constant2/1 -> Divide/2
  Divide/1 -> CS Modified PLL1/1
  Phase_Calc1/3(Phase c) -> [Ic_phase]
  Phase_Calc1/2(Phase b) -> [Ib_phase]
  Phase_Calc1/1(Phase a) -> [Ia_phase]
  [Iabc] -> Divide/1
  Phase_Calc/3(Phase c) -> [Vc_phase]
  Phase_Calc/2(Phase b) -> [Vb_phase]
  Phase_Calc/1(Phase a) -> [Va_phase]
  Gain2/1 -> CS Modified PLL/1
  [Vabc] -> Gain2/1
  [Q] -> Memory7/1
  [P] -> Memory5/1
  [pf] -> Gain1/1
  [freq] -> Gain4/1
  Bus Creator1/1 -> TO_MODBUS/1  "sm_in"
  FROM_MODBUS/1 -> Demux2/1
  [Vabc] -> Memory4/1
  [Iabc] -> Memory3/1
  Iabc/1 -> [Iabc]  "Iabc"
  [Vabc] -> PQ_Calculator/1(Vabc)
  [Iabc] -> PQ_Calculator/2(Iabc)
  [P] -> Gain10/1
  [Q] -> Gain6/1
  [S] -> Gain7/1
  [P] -> Apparent Power Power Factor/1
  [Q] -> Apparent Power Power Factor/2
  PQ_Calculator/1(P) -> [P]
  PQ_Calculator/2(Q) -> [Q]
  [Iabc] -> RMS_Calculator/1(Signal)
  [Vabc] -> RMS_Calculator1/1(Signal)
  RMS_Calculator/1(RMS_Signal) -> [Iabc_rms], Demux4/1
  RMS_Calculator1/1(RMS_Signal) -> [Vabc_rms], Demux5/1
  Demux4/3 -> [Ic_rms]
  Demux4/2 -> [Ib_rms]
  Demux4/1 -> [Ia_rms]
  Demux5/1 -> [Va_rms]
  Demux5/2 -> [Vb_rms]
  Demux5/3 -> [Vc_rms]
  Demux2/1 -> Fcn/1
  [Iabc] -> R50512759/1
  Demux2/2 -> [op_mode]

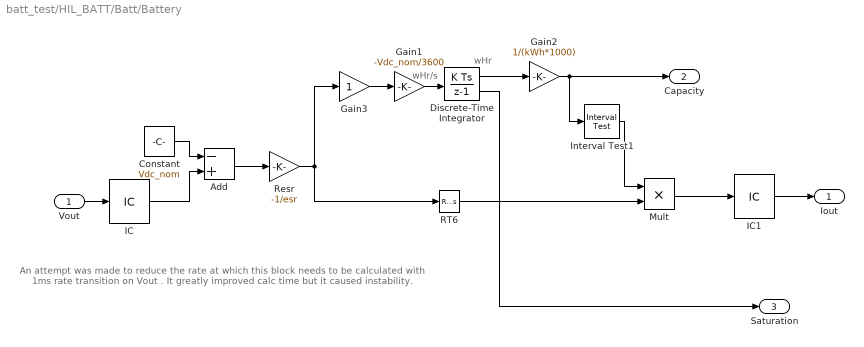
== system batt_test/HIL_BATT/Batt/Battery ==
  note: An attempt was made to reduce the rate at which this block
      | needs to be calculated with 1ms rate transition on
      | Vout .  It greatly improved calc time but it caused instability.
  note: wHr/s
  note: wHr
  Vout : Inport
  Add : Sum  Inputs=-+
  Constant : Constant  Value=Vdc_nom  SampleTime=Tds
  Discrete-Time Integrator : DiscreteIntegrator  InitialCondition=kWh*0.5*1000  InitialConditionMode=State only (most efficient)  SampleTime=Tds  LimitOutput=on  UpperSaturationLimit=(kWh*1000)  LowerSaturationLimit=0  ShowSaturationPort=on  ICPrevOutput=DiscIntNeverNeededParam  ICPrevScaledInput=DiscIntNeverNeededParam
  Gain1 : Gain  Gain=-Vdc_nom/3600
  Gain2 : Gain  Gain=1/(kWh*1000)
  Gain3 : Gain
  IC : InitialCondition  Value=Vdc_nom
  IC1 : InitialCondition  Value=0
  Interval Test1 : simulink/Logic and Bit Operations/Interval Test  IntervalClosedRight=on  uplimit=1  IntervalClosedLeft=on  lowlimit=0  OutDataTypeStr=boolean
  Mult : Product  Inputs=**
  RT6 : RateTransition  OutPortSampleTime=Tds
  Resr : Gain  Gain=-1/esr
  Iout : Outport
  Capacity : Outport  Port=2
  Saturation : Outport  Port=3
  wires:
  Constant/1 -> Add/1
  Add/1 -> Resr/1
  Gain1/1 -> Discrete-Time Integrator/1
  Interval Test1/1 -> Mult/1
  Vout/1 -> IC/1
  Mult/1 -> IC1/1
  Resr/1 -> RT6/1, Gain3/1
  Gain2/1 -> Capacity/1, Interval Test1/1
  Discrete-Time Integrator/1 -> Gain2/1
  IC/1 -> Add/2
  IC1/1 -> Iout/1
  RT6/1 -> Mult/2
  Gain3/1 -> Gain1/1
  Discrete-Time Integrator/2 -> Saturation/1

== system batt_test/HIL_BATT/Batt/Debounce1 ==
  In1 : Inport
  Compare To Constant1 : simulink/Logic and Bit Operations/Compare To Constant  relop=>  const=1  OutDataTypeStr=boolean
  Discrete-Time Integrator : DiscreteIntegrator  IntegratorMethod=Accumulation: Forward Euler  gainval=Ts/Td  ExternalReset=level  SampleTime=Ts  OutDataTypeStr=double  UpperSaturationLimit=1.001  LowerSaturationLimit=0  ICPrevOutput=DiscIntNeverNeededParam  ICPrevScaledInput=DiscIntNeverNeededParam
  Logical Operator : Logic  Operator=NOT  AllPortsSameDT=off  OutDataTypeStr=boolean
  Out1 : Outport
  wires:
  Compare To Constant1/1 -> Out1/1
  In1/1 -> Discrete-Time Integrator/1, Logical Operator/1
  Logical Operator/1 -> Discrete-Time Integrator/2
  Discrete-Time Integrator/1 -> Compare To Constant1/1

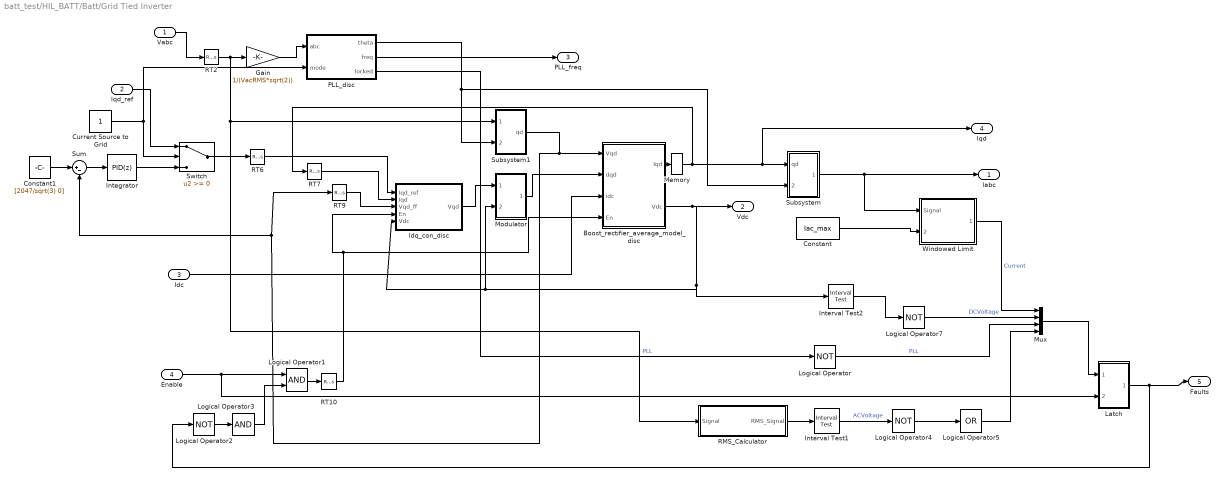
== system batt_test/HIL_BATT/Batt/Grid Tied Inverter ==
  Vabc : Inport
  Iqd_ref : Inport  Port=2
  Idc : Inport  Port=3
  Enable : Inport  Port=4
  Boost_rectifier_average_model_disc : Subsystem  mask{C=C, L=L, Roff=Roff, Vdc_nom=Vdc_nom}
      mask prompts: C "DC Bus Capacitance"; L "Boost Inductor"; Roff "Switch resistance when off"; Vdc_nom "Nominal DC Bus Voltage"
      mask init:
      | global_parameters
  Constant : Constant  Value=Iac_max
  Constant1 : Constant  Value=[2047/sqrt(3) 0]
  Current Source to Grid : Constant
  Gain : Gain  Gain=1/(VacRMS*sqrt(2))
  Idq_con_disc : Subsystem  mask{L=L, iq_max=Iq_at_max, id_max=Id_at_max, kp=I_kp, ki=I_ki, Vdc_nom=Vdc_nom}
      mask prompts: L "Boost Inductor"; iq_max "Maximum Iq"; id_max "Maximum Id"; kp "Proportional Gain"; ki "Integral Gain"; Vdc_nom "Nominal DC Bus Voltage"
      mask init:
      | global_parameters
  Integrator : simulink/Continuous/PID Controller  Controller=PID  TimeDomain=Discrete-time  SampleTime=Ts  IntegratorMethod=Forward Euler  FilterMethod=Forward Euler  Form=Parallel  P=2  I=0  D=0  N=100  InitialConditionSource=internal  InitialConditionForIntegrator=0  InitialConditionForFilter=0  ExternalReset=none  LimitOutput=on  UpperSaturationLimit=2000  LowerSaturationLimit=-2000  LinearizeAsGain=off  AntiWindupMode=clamping  Kb=1  TrackingMode=off  Kt=1  PParamMin=[]  PParamMax=[]  IParamMin=[]  IParamMax=[]  DParamMin=[]  DParamMax=[]  NParamMin=[]  NParamMax=[]  KbParamMin=[]  KbParamMax=[]  KtParamMin=[]  KtParamMax=[]  POutMin=[]  POutMax=[]  IOutMin=[]  IOutMax=[]  DOutMin=[]  DOutMax=[]  NOutMin=[]  NOutMax=[]  KbOutMin=[]  KbOutMax=[]  KtOutMin=[]  KtOutMax=[]  IntegratorOutMin=[]  IntegratorOutMax=[]  FilterOutMin=[]  FilterOutMax=[]  SumOutMin=[]  SumOutMax=[]  SumI1OutMin=[]  SumI1OutMax=[]  SumI2OutMin=[]  SumI2OutMax=[]  SumI3OutMin=[]  SumI3OutMax=[]  SumDOutMin=[]  SumDOutMax=[]  SaturationOutMin=[]  SaturationOutMax=[]  IntegratorContinuousStateAttributes=''  IntegratorStateMustResolveToSignalObject=off  IntegratorRTWStateStorageClass=Auto  FilterContinuousStateAttributes=''  FilterStateMustResolveToSignalObject=off  FilterRTWStateStorageClass=Auto
  Interval Test1 : simulink/Logic and Bit Operations/Interval Test  IntervalClosedRight=on  uplimit=VacRMS*1.1  IntervalClosedLeft=on  lowlimit=VacRMS*0.9  OutDataTypeStr=boolean
  Interval Test2 : simulink/Logic and Bit Operations/Interval Test  IntervalClosedRight=on  uplimit=Vdc_max  IntervalClosedLeft=on  lowlimit=2000  OutDataTypeStr=boolean
  Latch : Subsystem
  Logical Operator{,2,4,7} (4 alike) : Logic  Operator=NOT  AllPortsSameDT=off  OutDataTypeStr=boolean
  Logical Operator1 : Logic  AllPortsSameDT=off  OutDataTypeStr=boolean
  Logical Operator3 : Logic  Inputs=1  AllPortsSameDT=off  OutDataTypeStr=boolean
  Logical Operator5 : Logic  Operator=OR  Inputs=1  AllPortsSameDT=off  OutDataTypeStr=boolean
  Memory : Memory  InheritSampleTime=on
  Modulator : Subsystem
  Mux : Mux
  PLL_disc : Subsystem  mask{PLL_Kp=PLL_Kp, PLL_Ki=PLL_Ki, PLL_freq_range=0.25, PLL_lock_window=0.1}
      mask prompts: PLL_Kp "Proportional Gain"; PLL_Ki "Integral Gain"; PLL_freq_range "PLL Frequency Range"; PLL_lock_window "PLL Lock Window"
  RMS_Calculator : Subsystem
  RT{2,6..7,9..10} (5 alike) : RateTransition  OutPortSampleTime=Td_es_min
  Subsystem : Subsystem
  Subsystem1 : Subsystem
  Sum : Sum  Inputs=|+-
  Switch : Switch
  Windowed Limit : Subsystem
  Iabc : Outport
  Vdc : Outport  Port=2
  PLL_freq : Outport  Port=3
  Iqd : Outport  Port=4
  Faults : Outport  Port=5
  wires:
  Latch/1(Out1) -> Faults/1, Logical Operator2/1
  Mux/1 -> Latch/1(In1)
  RT7/1 -> Idq_con_disc/2(Iqd)
  Idc/1 -> Boost_rectifier_average_model_disc/3(idc)
  Boost_rectifier_average_model_disc/2(Vdc) -> Modulator/2(Vdc), Idq_con_disc/5(Vdc), Interval Test2/1, Vdc/1
  Logical Operator5/1 -> Mux/4
  Logical Operator4/1 -> Logical Operator5/1
  Interval Test1/1 -> Logical Operator4/1  "ACVoltage"
  RMS_Calculator/1(RMS_Signal) -> Interval Test1/1
  Logical Operator3/1 -> Logical Operator1/2
  Logical Operator2/1 -> Logical Operator3/1
  Subsystem1/1(qd) -> Boost_rectifier_average_model_disc/1(Vqd), RT9/1, Sum/2
  Boost_rectifier_average_model_disc/1(Iqd) -> Memory/1
  Subsystem/1(abc) -> Windowed Limit/1(Signal), Iabc/1
  Idq_con_disc/1(Vqd) -> Modulator/1(Vqd)
  Logical Operator1/1 -> RT10/1
  Constant/1 -> Windowed Limit/2(Threshold)
  Windowed Limit/1(TestOut) -> Mux/1  "Current"
  Interval Test2/1 -> Logical Operator7/1
  PLL_disc/2(freq) -> PLL_freq/1
  Modulator/1(dqd) -> Boost_rectifier_average_model_disc/2(dqd)
  PLL_disc/3(locked) -> Logical Operator/1  "PLL"
  Logical Operator/1 -> Mux/3  "PLL"
  Gain/1 -> PLL_disc/1(abc)
  Enable/1 -> Logical Operator1/1, Latch/2(Reset)
  PLL_disc/1(theta) -> Subsystem1/2(theta), Subsystem/2(theta)
  Vabc/1 -> RT2/1
  RT2/1 -> RMS_Calculator/1(Signal), Subsystem1/1(abc), Gain/1
  RT6/1 -> Idq_con_disc/1(Iqd_ref)
  RT9/1 -> Idq_con_disc/3(Vqd_ff)
  RT10/1 -> Boost_rectifier_average_model_disc/4(En), Idq_con_disc/4(En)
  Memory/1 -> Subsystem/1(qd), Iqd/1, RT7/1
  Logical Operator7/1 -> Mux/2  "DCVoltage"
  Switch/1 -> RT6/1
  Integrator/1 -> Switch/3
  Iqd_ref/1 -> Switch/1
  Current Source to Grid/1 -> Switch/2, PLL_disc/2(mode)
  Sum/1 -> Integrator/1
  Constant1/1 -> Sum/1

== system batt_test/HIL_BATT/Batt/Latch ==
  In1 : Inport
  Reset : Inport  Port=2
  Demux : Demux  Outputs=2
  Logical Operator6 : Logic  Operator=NOT  AllPortsSameDT=off  OutDataTypeStr=boolean
  Mux : Mux  Inputs=2
  S-R Flip-Flop : simulink_extras/Flip Flops/S-R Flip-Flop  initial_condition=0
  S-R Flip-Flop1 : simulink_extras/Flip Flops/S-R Flip-Flop  initial_condition=0
  Out1 : Outport
  wires:
  S-R Flip-Flop/1 -> Mux/1  "Ia"
  Mux/1 -> Out1/1  "Faults"
  Demux/1 -> S-R Flip-Flop/1
  In1/1 -> Demux/1
  S-R Flip-Flop1/1 -> Mux/2  "Ib"
  Demux/2 -> S-R Flip-Flop1/1
  Reset/1 -> Logical Operator6/1
  Logical Operator6/1 -> S-R Flip-Flop/2, S-R Flip-Flop1/2

== system batt_test/SEL_787_Relay1/SEL_787_Relay/PQ_Calculator ==
  Vabc : Inport
  Iabc : Inport  Port=2
  3-phase  Instantaneous  Active & Reactive Power : powerlib_extras/Measurements/3-phase  Instantaneous  Active & Reactive Power
  Demux : Demux  Outputs=2
  Discrete  Mean value2 : powerlib_extras/Discrete Measurements/Discrete  Mean value  Freq=60  Vinit=0  Ts=Ts
  P : Outport
  Q : Outport  Port=2
  wires:
  3-phase  Instantaneous  Active & Reactive Power/1 -> Discrete  Mean value2/1
  Discrete  Mean value2/1 -> Demux/1
  Vabc/1 -> 3-phase  Instantaneous  Active & Reactive Power/1
  Iabc/1 -> 3-phase  Instantaneous  Active & Reactive Power/2
  Demux/1 -> P/1  "P"
  Demux/2 -> Q/1  "Q"

== system batt_test/SEL_787_Relay1/SEL_787_Relay/Phase_Calc ==
  note: Assumes Ib and Ic are shifted 120 degrees from Ia
      | For accurate phase measurements, could use a single-
      | phase PLL for each phase
  wt : Inport
  Add2 : Sum  Inputs=+-
  Add3 : Sum
  Constant5 : Constant  Value=120
  Constant6 : Constant  Value=120
  Constant7 : Constant  Value=2*pi
  Constant8 : Constant  Value=2*pi
  Math Function : Math  Operator=mod  SaturateOnIntegerOverflow=on
  Math Function1 : Math  Operator=mod  SaturateOnIntegerOverflow=on
  Phase a : Outport
  Phase b : Outport  Port=2
  Phase c : Outport  Port=3
  wires:
  Math Function1/1 -> Phase c/1
  Math Function/1 -> Phase b/1
  Constant8/1 -> Math Function1/2
  Add3/1 -> Math Function1/1
  Add2/1 -> Math Function/1
  Constant7/1 -> Math Function/2
  wt/1 -> Add3/1, Phase a/1, Add2/1
  Constant6/1 -> Add3/2
  Constant5/1 -> Add2/2

== system batt_test/SEL_787_Relay1/SEL_787_Relay/Phase_Calc1 ==
  note: Assumes Ib and Ic are shifted 120 degrees from Ia
      | For accurate phase measurements, could use a single-
      | phase PLL for each phase
  wt : Inport
  Add2 : Sum  Inputs=+-
  Add3 : Sum
  Constant5 : Constant  Value=120
  Constant6 : Constant  Value=120
  Constant7 : Constant  Value=2*pi
  Constant8 : Constant  Value=2*pi
  Math Function : Math  Operator=mod  SaturateOnIntegerOverflow=on
  Math Function1 : Math  Operator=mod  SaturateOnIntegerOverflow=on
  Phase a : Outport
  Phase b : Outport  Port=2
  Phase c : Outport  Port=3
  wires:
  Constant5/1 -> Add2/2
  Constant6/1 -> Add3/2
  wt/1 -> Add2/1, Phase a/1, Add3/1
  Constant7/1 -> Math Function/2
  Add2/1 -> Math Function/1
  Add3/1 -> Math Function1/1
  Constant8/1 -> Math Function1/2
  Math Function/1 -> Phase b/1
  Math Function1/1 -> Phase c/1

== system batt_test/SEL_787_Relay1/SEL_787_Relay/RMS_Calculator ==
  Signal : Inport
  Discrete  Mean value6 : powerlib_extras/Discrete Measurements/Discrete  Mean value  Freq=60  Vinit=0  Ts=Ts
  Product3 : Product  RndMeth=Zero
  Signed Sqrt : Sqrt  SaturateOnIntegerOverflow=on
  RMS_Signal : Outport
  wires:
  Signal/1 -> Product3/1, Product3/2
  Product3/1 -> Discrete  Mean value6/1
  Discrete  Mean value6/1 -> Signed Sqrt/1
  Signed Sqrt/1 -> RMS_Signal/1

== system batt_test/SEL_787_Relay1/SEL_787_Relay/RMS_Calculator1 ==
  Signal : Inport
  Discrete  Mean value6 : powerlib_extras/Discrete Measurements/Discrete  Mean value  Freq=60  Vinit=0  Ts=Ts
  Product3 : Product  RndMeth=Zero
  Signed Sqrt : Sqrt  SaturateOnIntegerOverflow=on
  RMS_Signal : Outport
  wires:
  Signal/1 -> Product3/1, Product3/2
  Product3/1 -> Discrete  Mean value6/1
  Discrete  Mean value6/1 -> Signed Sqrt/1
  Signed Sqrt/1 -> RMS_Signal/1

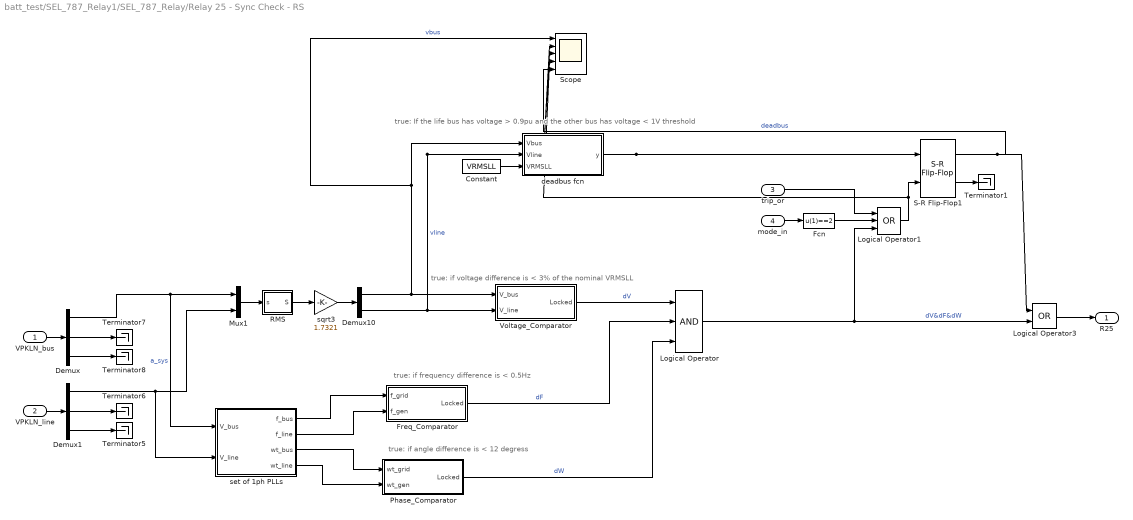
== system batt_test/SEL_787_Relay1/SEL_787_Relay/Relay 25 - Sync Check - RS ==
  note: true: if angle difference is < 12 degress
  note: true: if frequency difference is < 0.5Hz
  note: true: if voltage difference is < 3% of the nominal VRMSLL
  note: true: If the life bus has voltage > 0.9pu and the other bus has voltage < 1V threshold
  VPKLN_bus : Inport
  VPKLN_line : Inport  Port=2
  trip_or : Inport  Port=3
  mode_in : Inport  Port=4
  Constant : Constant  Value=VRMSLL
  Demux : Demux  Outputs=3
  Demux1 : Demux  Outputs=3
  Demux10 : Demux  Outputs=2
  Fcn : Fcn  Expr=u(1)==2
  Freq_Comparator : Subsystem
  Logical Operator : Logic  Inputs=3  AllPortsSameDT=off  OutDataTypeStr=boolean
  Logical Operator1 : Logic  Operator=OR  Inputs=3  AllPortsSameDT=off  OutDataTypeStr=boolean
  Logical Operator3 : Logic  Operator=OR  AllPortsSameDT=off  OutDataTypeStr=boolean
  Mux1 : Mux  Inputs=2
  Phase_Comparator : Subsystem
  RMS : Subsystem
  S-R Flip-Flop1 : simulink_extras/Flip Flops/S-R Flip-Flop  initial_condition=0
  Scope : Scope  NumInputPorts=5
      settings: YMin=0~0~-1~0.95~-5  YMax=2250~3000~1~1.05~5  SaveName=ScopeData5
  Terminator{1,5..8} (5 alike) : Terminator
  Voltage_Comparator : Subsystem
  deadbus fcn : MATLAB Function  TreatAsAtomicUnit=on
  set of 1ph PLLs : Subsystem
  sqrt3 : Gain  Gain=1.7321
  R25 : Outport
  wires:
  Fcn/1 -> Logical Operator1/2
  mode_in/1 -> Fcn/1
  trip_or/1 -> Logical Operator1/1
  Logical Operator1/1 -> S-R Flip-Flop1/2, Scope/4
  deadbus fcn/1(y) -> S-R Flip-Flop1/1, Scope/3
  S-R Flip-Flop1/1 -> Logical Operator3/1, Scope/5  "deadbus"
  Logical Operator3/1 -> R25/1
  S-R Flip-Flop1/2 -> Terminator1/1
  Constant/1 -> deadbus fcn/3(VRMSLL)
  sqrt3/1 -> Demux10/1
  Mux1/1 -> RMS/1(s)
  RMS/1(S) -> sqrt3/1
  Phase_Comparator/1(Locked) -> Logical Operator/3  "dW"
  Freq_Comparator/1(Locked) -> Logical Operator/2  "dF"
  Voltage_Comparator/1(Locked) -> Logical Operator/1  "dV"
  Demux10/2 -> Voltage_Comparator/2(V_line), deadbus fcn/2(Vline), Scope/2  "vline"
  set of 1ph PLLs/4(wt_line) -> Phase_Comparator/2(wt_gen)
  set of 1ph PLLs/3(wt_bus) -> Phase_Comparator/1(wt_grid)
  set of 1ph PLLs/2(f_line) -> Freq_Comparator/2(f_gen)
  set of 1ph PLLs/1(f_bus) -> Freq_Comparator/1(f_grid)
  Demux10/1 -> Voltage_Comparator/1(V_bus), deadbus fcn/1(Vbus), Scope/1  "vbus"
  Demux/1 -> Mux1/1, set of 1ph PLLs/1(V_bus)  "a_sys"
  Demux1/1 -> Mux1/2, set of 1ph PLLs/2(V_line)
  Demux1/2 -> Terminator6/1
  Demux1/3 -> Terminator5/1
  Demux/2 -> Terminator7/1
  Demux/3 -> Terminator8/1
  VPKLN_bus/1 -> Demux/1
  VPKLN_line/1 -> Demux1/1
  Logical Operator/1 -> Logical Operator1/3, Logical Operator3/2  "dV&dF&dW"
